simulink model "arm_stereo_ibvs_ekf_v1"  (R2025b)
settings: Solver=FixedStepDiscrete  StartTime=0  StopTime=inf  FixedStep=cfg.Ts  RelTol=1e-3
InitFcn:
  | init_arm_stereo_ibvs_ekf_v1
values from neighbouring files (symbols this model uses):
  cfg = cfgOverrideLocal    [init_arm_stereo_ibvs_ekf_v1.m]
  data = Stateflow.Data(chart)    [build_arm_stereo_ibvs_ekf_v1.m]
undefined symbols (not defined in the file or in its folder): cfg_armDepthRampTime, cfg_baseline, cfg_betaC, cfg_betaRho, cfg_cartesianLinearSpeedMax, cfg_cxL, cfg_cxR, cfg_cyL, cfg_cyR, cfg_disparityMin, cfg_disturbanceConfirmTime, cfg_ekfCovarianceJitter, cfg_ekfP0, cfg_ekfSConditionMin, cfg_ekfX0, cfg_epsilonC, cfg_epsilonRho, cfg_focalLength0Mm, cfg_focalLengthHardwareMaxMm, cfg_focalLengthHardwareMinMm, cfg_focalLengthWorkingMaxMm, cfg_focalLengthWorkingMinMm, cfg_focalRateAbsoluteMaxMmPerSec, cfg_focalRateGuaranteedMmPerSec, cfg_fr3Axis, cfg_fr3Joint8OriginRPY, cfg_fr3Joint8OriginXYZ, cfg_fr3OriginRPY, cfg_fr3OriginXYZ, cfg_imageWidth, cfg_Kc, cfg_kRho, cfg_lambdaC, cfg_lambdaRho, cfg_numericalEpsilon, cfg_outputPixelPitchXmm, cfg_outputPixelPitchYmm, cfg_p_CL_CR, cfg_pixelNoiseStd, cfg_q0, cfg_R_CL_CR, cfg_rhoMax, cfg_rhoMin, cfg_rightVisibilityHysteresisPx, cfg_rightVisibilityMarginPx, cfg_robustEnable, cfg_ros2InputTimeoutSec, cfg_scaleErrorEnterThreshold, cfg_scaleErrorExitThreshold, cfg_scaleSettledHoldTime, cfg_sigmaJerk, cfg_T_CL_CR, cfg_T_link8_CL, cfg_T_W_B, cfg_targetCharacteristicSize, cfg_Ts, cfg_visibilityEpsilon, cfg_visibilityZMin, cfg_zoomLimitMarginFraction, cfg_zoomOnlyMaxTime ... (+2)
libraries: ros2lib x7
(part 2 of 2)

== matlab function arm_stereo_ibvs_ekf_v1/Arm Priority Controller/MATLAB Function ==
  data: cameraVelocityCmd output; cLMeasured input; rhoHatL input; vHatLeft input; cLd input; rhoD input; validLeft input; ekfPredictionValid input; centerEnable input; depthEnable input; armEnable input; depthTaskWeight input; centerError output; depthError output; centerConditionMetric output; depthAuthority output; cameraVelocityCenter output; cameraVelocityDepthRaw output; cameraVelocityDepthWeighted output; cfg_numericalEpsilon parameter double size=[1 1]; cfg_robustEnable parameter double size=[1 1]; cfg_betaC parameter double size=[1 1]; cfg_epsilonC parameter double size=[1 1]; cfg_Kc parameter double size=[2 2]; cfg_lambdaC parameter double size=[1 1]; cfg_betaRho parameter double size=[1 1]; cfg_epsilonRho parameter double size=[1 1]; cfg_kRho parameter double size=[1 1]; cfg_lambdaRho parameter double size=[1 1]
function [cameraVelocityCmd, ...
          centerError, ...
          depthError, ...
          centerConditionMetric, ...
          depthAuthority, ...
          cameraVelocityCenter, ...
          cameraVelocityDepthRaw, ...
          cameraVelocityDepthWeighted] = fcn( ...
          cLMeasured, ...
          rhoHatL, ...
          vHatLeft, ...
          cLd, ...
          rhoD, ...
          validLeft, ...
          ekfPredictionValid, ...
          centerEnable, ...
          depthEnable, ...
          armEnable, ...
          depthTaskWeight, ...
          cfg_numericalEpsilon, ...
          cfg_robustEnable, ...
          cfg_betaC, ...
          cfg_epsilonC, ...
          cfg_Kc, ...
          cfg_lambdaC, ...
          cfg_betaRho, ...
          cfg_epsilonRho, ...
          cfg_kRho, ...
          cfg_lambdaRho)
%#codegen
% 输出均为左相机坐标系下的6维相机速度：
% [vx; vy; vz; wx; wy; wz]
%
% 中心任务为主任务，逆深度任务在中心任务零空间中执行。
% 关节速度映射、关节零空间和关节安全由外部ROS节点负责。

cameraVelocityCmd           = zeros(6,1);
centerError                 = zeros(2,1);
depthError                  = 0;
centerConditionMetric       = 0;
depthAuthority              = 0;
cameraVelocityCenter        = zeros(6,1);
cameraVelocityDepthRaw      = zeros(6,1);
cameraVelocityDepthWeighted = zeros(6,1);

%% 1. 基本安全门控
if armEnable <= 0.5 || validLeft <= 0.5
    return;
end

x = cLMeasured(1);
y = cLMeasured(2);

if ~isfinite(x) || ~isfinite(y)
    return;
end

%% 2. 选择逆深度和目标速度前馈
rho = max(rhoD, cfg_numericalEpsilon);
vFeed = zeros(3,1);

if ekfPredictionValid > 0.5 && ...
        isfinite(rhoHatL) && rhoHatL > cfg_numericalEpsilon && ...
        all(isfinite(vHatLeft))

    rho = max(rhoHatL, cfg_numericalEpsilon);
    vFeed = vHatLeft;
end

%% 3. 左相机中心任务
centerError = [x; y] - cLd;

Lc = [ ...
    -rho,  0,     x*rho, x*y,     -(1+x*x),  y;
     0,   -rho,   y*rho, 1+y*y,   -x*y,     -x];

Hc = rho * [ ...
    1, 0, -x;
    0, 1, -y];

bHatC = Hc * vFeed;

robustCenter = zeros(2,1);

if cfg_robustEnable > 0.5
    robustCenter = cfg_betaC * centerError / ...
        (sqrt(centerError' * centerError) + cfg_epsilonC);
end

nuCenter = -cfg_Kc * centerError ...
           -bHatC ...
           -robustCenter;

Gc = Lc * Lc' + cfg_lambdaC^2 * eye(2);
LcDampedInverse = Lc' / Gc;

cameraVelocityCenter = LcDampedInverse * nuCenter;

% 中心任务零空间
Ncenter = eye(6) - LcDampedInverse * Lc;

% 仅作为诊断值，越接近0说明中心任务数值条件越差
centerConditionMetric = det(Gc) / ...
    (trace(Gc)^2 + cfg_numericalEpsilon);

%% 4. 逆深度任务
depthError = rho - rhoD;

Lrho = [0, 0, rho*rho, rho*y, -rho*x, 0];
Hrho = [0, 0, -rho*rho];

bHatRho = Hrho * vFeed;

robustDepth = 0;

if cfg_robustEnable > 0.5
    robustDepth = cfg_betaRho * depthError / ...
        (abs(depthError) + cfg_epsilonRho);
end

nuDepth = -cfg_kRho * depthError ...
          -bHatRho ...
          -robustDepth;

% 深度任务在中心任务零空间中的有效方向
Adepth = Lrho * Ncenter;

depthAuthority = Adepth * Adepth';
depthDenominator = depthAuthority + cfg_lambdaRho^2;

depthWeight = min(max(depthTaskWeight, 0), 1);

if ekfPredictionValid <= 0.5
    depthWeight = 0;
end

cameraVelocityDepthRaw = ...
    Ncenter * Adepth' * ...
    ((nuDepth - Lrho * cameraVelocityCenter) / depthDenominator);

cameraVelocityDepthWeighted = ...
    depthWeight * cameraVelocityDepthRaw;

%% 5. 组合控制命令
if centerEnable > 0.5
    cameraVelocityCmd = cameraVelocityCenter;
end

if depthEnable > 0.5 && ekfPredictionValid > 0.5

    if centerEnable > 0.5
        % 中心主任务 + 深度零空间次任务
        cameraVelocityCmd = ...
            cameraVelocityCenter + cameraVelocityDepthWeighted;
    else
        % 仅执行深度任务
        standaloneDenominator = ...
            Lrho * Lrho' + cfg_lambdaRho^2;

        cameraVelocityDepthRaw = ...
            Lrho' * (nuDepth / standaloneDenominator);

        cameraVelocityDepthWeighted = ...
            depthWeight * cameraVelocityDepthRaw;

        cameraVelocityCenter = zeros(6,1);
        cameraVelocityCmd = cameraVelocityDepthWeighted;
    end
end

%% 6. 数值安全
if any(~isfinite(cameraVelocityCmd))
    cameraVelocityCmd = zeros(6,1);
end

if any(~isfinite(cameraVelocityCenter))
    cameraVelocityCenter = zeros(6,1);
end

if any(~isfinite(cameraVelocityDepthRaw))
    cameraVelocityDepthRaw = zeros(6,1);
end

if any(~isfinite(cameraVelocityDepthWeighted))
    cameraVelocityDepthWeighted = zeros(6,1);
end
end

== matlab function arm_stereo_ibvs_ekf_v1/Estimated Rho Dynamics/MATLAB Function ==
  data: normalizedFeatureMeasured input; rhoDotHat output; rhoHat input; vHatCL input; vHatCR input; JL input; JR input; qDotApplied input; cfg_R_CL_CR parameter double size=[3 3]; cfg_p_CL_CR parameter double size=[3 1]; cfg_numericalEpsilon parameter double size=[1 1]
function rhoDotHat = fcn(normalizedFeatureMeasured,rhoHat,vHatCL,vHatCR,JL,JR,qDotApplied, cfg_R_CL_CR, cfg_p_CL_CR, cfg_numericalEpsilon)
%#codegen
% Predicted inverse-depth rate from the applied left-camera twist.
rhoDotHat=zeros(2,1);
VCL=reshape(qDotApplied,6,1); R=cfg_R_CL_CR; p=cfg_p_CL_CR; S=[0 -p(3) p(2);p(3) 0 -p(1);-p(2) p(1) 0]; VCR=[R' -R'*S;zeros(3,3) R']*VCL;
for i=1:2
    if i==1, x=normalizedFeatureMeasured(1); y=normalizedFeatureMeasured(2); rho=max(rhoHat,cfg_numericalEpsilon); Vcam=VCL; vt=vHatCL;
    else, x=normalizedFeatureMeasured(3); y=normalizedFeatureMeasured(4); rho=max(rhoHat,cfg_numericalEpsilon); Vcam=VCR; vt=vHatCR; end
    Lrho=[0 0 rho*rho rho*y -rho*x 0]; Hrho=[0 0 -rho*rho];
    rhoDotHat(i)=Lrho*Vcam+Hrho*vt;
end
rhoDotHat=rhoDotHat+0*sum(JL(:))+0*sum(JR(:));
if any(~isfinite(rhoDotHat)), rhoDotHat=zeros(2,1); end
end

== matlab function arm_stereo_ibvs_ekf_v1/Right Visibility Guard/MATLAB Function ==
  data: xLeftMeasured input; uRightPredicted output; rhoHatSafe input; focalLengthMeasuredMm input; validLeft input; validRight input; ekfPredictionValid input; rightReacquireActive input; scaleDesiredNominal input; reset input; rightVisibilityMarginActualPx output; fRightMaxVisibleMm output; fRightMaxEffectiveMm output; rightScaleDesiredEffective output; rightVisibilityActive output; rightVisibilityInfeasible output; scaleDesiredEffective output; rightScaleDesiredNominal output; fRightMeasuredMm output; cfg_numericalEpsilon parameter double size=[1 1]; cfg_baseline parameter double size=[1 1]; cfg_outputPixelPitchXmm parameter double size=[1 1]; cfg_cxR parameter double size=[1 1]; cfg_imageWidth parameter double size=[1 1]; cfg_focalLengthHardwareMaxMm parameter double size=[2 1]; cfg_visibilityEpsilon parameter double size=[1 1]; cfg_rightVisibilityMarginPx parameter double size=[1 1]; cfg_focalLengthWorkingMaxMm parameter double size=[2 1]; cfg_focalLengthWorkingMinMm parameter double size=[2 1]; cfg_targetCharacteristicSize parameter double size=[1 1]; cfg_rightVisibilityHysteresisPx parameter double size=[1 1]
function [uRightPredicted,rightVisibilityMarginActualPx,fRightMaxVisibleMm,fRightMaxEffectiveMm,rightScaleDesiredEffective,rightVisibilityActive,rightVisibilityInfeasible,scaleDesiredEffective,rightScaleDesiredNominal,fRightMeasuredMm] = fcn(xLeftMeasured,rhoHatSafe,focalLengthMeasuredMm,validLeft,validRight,ekfPredictionValid,rightReacquireActive,scaleDesiredNominal,reset, cfg_numericalEpsilon, cfg_baseline, cfg_outputPixelPitchXmm, cfg_cxR, cfg_imageWidth, cfg_focalLengthHardwareMaxMm, cfg_visibilityEpsilon, cfg_rightVisibilityMarginPx, cfg_focalLengthWorkingMaxMm, cfg_focalLengthWorkingMinMm, cfg_targetCharacteristicSize, cfg_rightVisibilityHysteresisPx)
%#codegen
% CURRENT_STATE_VISIBILITY_GUARD; interface retained for future one-step prediction.
persistent active
if isempty(active), active=1; end
if reset>0.5, active=1; end
rightScaleDesiredNominal=scaleDesiredNominal(2); fRightMeasuredMm=focalLengthMeasuredMm(2); rho=max(rhoHatSafe,cfg_numericalEpsilon); xR=xLeftMeasured-cfg_baseline*rho; fRightPx=focalLengthMeasuredMm(2)/cfg_outputPixelPitchXmm;
uRightPredicted=cfg_cxR+fRightPx*xR; rightVisibilityMarginActualPx=min(uRightPredicted,cfg_imageWidth-uRightPredicted);
hardwareMaxPx=cfg_focalLengthHardwareMaxMm(2)/cfg_outputPixelPitchXmm;
if xR < -cfg_visibilityEpsilon, fMaxPx=(cfg_cxR-cfg_rightVisibilityMarginPx)/(-xR); elseif xR > cfg_visibilityEpsilon, fMaxPx=(cfg_imageWidth-cfg_rightVisibilityMarginPx-cfg_cxR)/xR; else, fMaxPx=hardwareMaxPx; end
fMaxPx=max(fMaxPx,0); fRightMaxVisibleMm=fMaxPx*cfg_outputPixelPitchXmm; rawEffective=min([cfg_focalLengthWorkingMaxMm(2);cfg_focalLengthHardwareMaxMm(2);fRightMaxVisibleMm]);
rightVisibilityInfeasible=double(rawEffective<cfg_focalLengthWorkingMinMm(2)); fRightMaxEffectiveMm=max(cfg_focalLengthWorkingMinMm(2),rawEffective);
scaleRightMaxVisible=cfg_targetCharacteristicSize*fMaxPx*rho; rightScaleDesiredEffective=min(scaleDesiredNominal(2),max(scaleRightMaxVisible,cfg_numericalEpsilon)); scaleDesiredEffective=[scaleDesiredNominal(1);rightScaleDesiredEffective];
enter=(validLeft<=0.5)||(ekfPredictionValid<=0.5)||(validRight<=0.5)||(rightReacquireActive>0.5)||(rightVisibilityInfeasible>0.5)||(uRightPredicted<cfg_rightVisibilityMarginPx)||(uRightPredicted>cfg_imageWidth-cfg_rightVisibilityMarginPx)||(focalLengthMeasuredMm(2)>fRightMaxEffectiveMm+cfg_numericalEpsilon);
exitOK=validLeft>0.5&&validRight>0.5&&ekfPredictionValid>0.5&&rightReacquireActive<=0.5&&rightVisibilityInfeasible<=0.5&&uRightPredicted>=cfg_rightVisibilityMarginPx+cfg_rightVisibilityHysteresisPx&&uRightPredicted<=cfg_imageWidth-cfg_rightVisibilityMarginPx-cfg_rightVisibilityHysteresisPx&&focalLengthMeasuredMm(2)<=fRightMaxEffectiveMm;
if enter, active=1; elseif exitOK, active=0; end; rightVisibilityActive=double(active>0.5);
if any(~isfinite([uRightPredicted;rightVisibilityMarginActualPx;fRightMaxVisibleMm;fRightMaxEffectiveMm;rightScaleDesiredEffective])), uRightPredicted=cfg_cxR; rightVisibilityMarginActualPx=0; fRightMaxVisibleMm=0; fRightMaxEffectiveMm=cfg_focalLengthWorkingMinMm(2); rightScaleDesiredEffective=cfg_numericalEpsilon; scaleDesiredEffective=[scaleDesiredNominal(1);rightScaleDesiredEffective]; rightVisibilityActive=1; rightVisibilityInfeasible=1; end
end

== matlab function arm_stereo_ibvs_ekf_v1/Zoom Controller/MATLAB Function ==
  data: fMeasuredMm input; fDotMmCmd output; scaleMeasured input; rhoHat input; rhoDotHat input; scaleDesiredEffective input; validLeft input; ekfPredictionValid input; focalAtWorkingLowerLimit input; focalAtWorkingUpperLimit input; fRightMaxEffectiveMm input; rightVisibilityActive input; rightReacquireActive input; fDotMmLimited output; scaleError output; gDotCmd output; focalCommandOutwardAtWorkingLimit output; focalFeasible output; focalRateUsageGuaranteedCmd output; focalRateUsageHardCmd output; cfg_focalLengthWorkingMaxMm parameter double size=[2 1]; cfg_numericalEpsilon parameter double size=[1 1]; cfg_robustEnable parameter double size=[1 1]; cfg_betaF parameter double size=[2 1]; cfg_epsilonF parameter double size=[2 1]; cfg_Kf parameter double size=[2 2]; cfg_targetCharacteristicSize parameter double size=[1 1]; cfg_outputPixelPitchXmm parameter double size=[1 1]; cfg_focalLengthWorkingMinMm parameter double size=[2 1]; cfg_rightReacquireZoomRateMmPerSec parameter double size=[1 1]; cfg_focalRateDesignMmPerSec parameter double size=[1 1]; cfg_Ts parameter double size=[1 1]; cfg_focalRateGuaranteedMmPerSec parameter double size=[1 1]; cfg_focalRateAbsoluteMaxMmPerSec parameter double size=[1 1]; cfg_zoomControlEnable parameter double size=[1 1]
function [fDotMmCmd,fDotMmLimited,scaleError,gDotCmd,focalCommandOutwardAtWorkingLimit,focalFeasible,focalRateUsageGuaranteedCmd,focalRateUsageHardCmd] = fcn(fMeasuredMm,scaleMeasured,rhoHat,rhoDotHat,scaleDesiredEffective,validLeft,ekfPredictionValid,focalAtWorkingLowerLimit,focalAtWorkingUpperLimit,fRightMaxEffectiveMm,rightVisibilityActive,rightReacquireActive, cfg_focalLengthWorkingMaxMm, cfg_numericalEpsilon, cfg_robustEnable, cfg_betaF, cfg_epsilonF, cfg_Kf, cfg_targetCharacteristicSize, cfg_outputPixelPitchXmm, cfg_focalLengthWorkingMinMm, cfg_rightReacquireZoomRateMmPerSec, cfg_focalRateDesignMmPerSec, cfg_Ts, cfg_focalRateGuaranteedMmPerSec, cfg_focalRateAbsoluteMaxMmPerSec, cfg_zoomControlEnable)
%#codegen
% Independent log-focal-length control; focal length is measured, not estimated.
fDotMmCmd=zeros(2,1); fDotMmLimited=zeros(2,1); scaleError=zeros(2,1); gDotCmd=zeros(2,1); focalCommandOutwardAtWorkingLimit=zeros(2,1); focalFeasible=ones(2,1); focalRateUsageGuaranteedCmd=zeros(2,1); focalRateUsageHardCmd=zeros(2,1);
upperEffective=[cfg_focalLengthWorkingMaxMm(1);fRightMaxEffectiveMm]; rho=max(rhoHat,cfg_numericalEpsilon);
for i=1:2
    r=max(scaleMeasured(i),cfg_numericalEpsilon); rd=max(scaleDesiredEffective(i),cfg_numericalEpsilon);
    scaleError(i)=log(r/rd); dHat=rhoDotHat(i)/rho; rf=0;
    if cfg_robustEnable>0.5, rf=cfg_betaF(i)*scaleError(i)/(abs(scaleError(i))+cfg_epsilonF(i)); end
    gDotCmd(i)=-cfg_Kf(i,i)*scaleError(i)-dHat-rf; fDotMmCmd(i)=fMeasuredMm(i)*gDotCmd(i);
    fRequiredMm=scaleDesiredEffective(i)/(cfg_targetCharacteristicSize*rho)*cfg_outputPixelPitchXmm; if fRequiredMm<cfg_focalLengthWorkingMinMm(i)||fRequiredMm>upperEffective(i), focalFeasible(i)=0; end
    focalCommandOutwardAtWorkingLimit(i)=double((focalAtWorkingLowerLimit(i)>0.5&&fDotMmCmd(i)<0)||(focalAtWorkingUpperLimit(i)>0.5&&fDotMmCmd(i)>0)||(fMeasuredMm(i)>=upperEffective(i)&&fDotMmCmd(i)>0));
end
if rightVisibilityActive>0.5||rightReacquireActive>0.5, if fMeasuredMm(2)>fRightMaxEffectiveMm+cfg_numericalEpsilon, fDotMmCmd(2)=-cfg_rightReacquireZoomRateMmPerSec; else, fDotMmCmd(2)=min(fDotMmCmd(2),0); end; end
if validLeft<=0.5||ekfPredictionValid<=0.5, fDotMmCmd(1)=0; if fMeasuredMm(1)>cfg_focalLengthWorkingMinMm(1), fDotMmCmd(1)=-cfg_rightReacquireZoomRateMmPerSec; end; fDotMmCmd(2)=0; if fMeasuredMm(2)>cfg_focalLengthWorkingMinMm(2), fDotMmCmd(2)=-cfg_rightReacquireZoomRateMmPerSec; end; end
fDotMmLimited=min(max(fDotMmCmd,-cfg_focalRateDesignMmPerSec),cfg_focalRateDesignMmPerSec); nextRight=fMeasuredMm(2)+cfg_Ts*fDotMmLimited(2); if fMeasuredMm(2)<=fRightMaxEffectiveMm&&nextRight>fRightMaxEffectiveMm, fDotMmLimited(2)=min(fDotMmLimited(2),(fRightMaxEffectiveMm-fMeasuredMm(2))/cfg_Ts); end
focalRateUsageGuaranteedCmd=abs(fDotMmLimited)/cfg_focalRateGuaranteedMmPerSec; focalRateUsageHardCmd=abs(fDotMmLimited)/cfg_focalRateAbsoluteMaxMmPerSec;
if cfg_zoomControlEnable<=0.5 || any(~isfinite(fDotMmCmd))||any(~isfinite(fDotMmLimited)), fDotMmCmd=zeros(2,1); fDotMmLimited=zeros(2,1); gDotCmd=zeros(2,1); focalRateUsageGuaranteedCmd=zeros(2,1); focalRateUsageHardCmd=zeros(2,1); end
end

== matlab function arm_stereo_ibvs_ekf_v1/Zoom Priority Supervisor/MATLAB Function ==
  data: scaleError input; depthTaskWeight output; depthError input; focalLengthMeasuredMm input; focalAtWorkingLowerLimit input; focalAtWorkingUpperLimit input; focalHeadroomMm input; focalFeasible input; validLeft input; validStereoQualified input; ekfPredictionValid input; reset input; focalCommandOutwardAtWorkingLimit input; focalRateUsageGuaranteed input; focalRateUsageHard input; rightReacquireActive input; schedulerMode output; zoomPriorityActive output; zoomPriorityTimer output; scaleSettledTimer output; armRecoveryReason output; newDisturbanceDetected output; cfg_zoomPriorityEnable parameter double size=[1 1]; cfg_armDepthRampTime parameter double size=[1 1]; cfg_scaleErrorEnterThreshold parameter double size=[1 1]; cfg_Ts parameter double size=[1 1]; cfg_scaleErrorExitThreshold parameter double size=[1 1]; cfg_disturbanceConfirmTime parameter double size=[1 1]; cfg_scaleSettledHoldTime parameter double size=[1 1]; cfg_zoomOnlyMaxTime parameter double size=[1 1]
function [depthTaskWeight,schedulerMode,zoomPriorityActive,zoomPriorityTimer,scaleSettledTimer,armRecoveryReason,newDisturbanceDetected]=fcn(scaleError,depthError,focalLengthMeasuredMm,focalAtWorkingLowerLimit,focalAtWorkingUpperLimit,focalHeadroomMm,focalFeasible,validLeft,validStereoQualified,ekfPredictionValid,reset,focalCommandOutwardAtWorkingLimit,focalRateUsageGuaranteed,focalRateUsageHard,rightReacquireActive, cfg_zoomPriorityEnable, cfg_armDepthRampTime, cfg_scaleErrorEnterThreshold, cfg_Ts, cfg_scaleErrorExitThreshold, cfg_disturbanceConfirmTime, cfg_scaleSettledHoldTime, cfg_zoomOnlyMaxTime)
%#codegen
% Modes: 0 INITIALIZE, 1 ZOOM_FIRST, 2 ARM_RECOVERY, 3 FULL_TRACK, 4 SAFE_HOLD, 5 RIGHT_REACQUIRE.
persistent mode zoomTimer settledTimer rampTimer reason disturbanceTimer validLast rateTimer
if isempty(mode), mode=0; zoomTimer=0; settledTimer=0; rampTimer=0; reason=0; disturbanceTimer=0; validLast=0; rateTimer=0; end
if reset>0.5, mode=0; zoomTimer=0; settledTimer=0; rampTimer=0; reason=0; disturbanceTimer=0; validLast=0; rateTimer=0; end
depthTaskWeight=0; newDisturbanceDetected=0; centerValid=validLeft>0.5; depthReady=validStereoQualified>0.5&&ekfPredictionValid>0.5&&rightReacquireActive<=0.5; e=max(abs(scaleError));
if ~centerValid, mode=4; depthTaskWeight=0; validLast=0;
elseif ~depthReady, mode=5; depthTaskWeight=0; validLast=0; rampTimer=0;
elseif cfg_zoomPriorityEnable<=0.5, mode=3; depthTaskWeight=1; zoomTimer=0; settledTimer=0; rampTimer=cfg_armDepthRampTime; reason=0; disturbanceTimer=0; validLast=1;
else
    if validLast<0.5&&(mode==4||mode==5), mode=1; zoomTimer=0; settledTimer=0; rampTimer=0; reason=0; disturbanceTimer=0; end
    if mode==0, if e>cfg_scaleErrorEnterThreshold, mode=1; depthTaskWeight=0; else, mode=3; depthTaskWeight=1; end
    elseif mode==1
        depthTaskWeight=0; zoomTimer=zoomTimer+cfg_Ts; if e<=cfg_scaleErrorExitThreshold, settledTimer=settledTimer+cfg_Ts; else, settledTimer=0; end
        if any(focalRateUsageGuaranteed>=1), rateTimer=rateTimer+cfg_Ts; else, rateTimer=0; end
        if any(focalRateUsageHard>=1), mode=2; reason=6; rampTimer=0;
        elseif rateTimer>=cfg_disturbanceConfirmTime&&e>cfg_scaleErrorExitThreshold, mode=2; reason=5; rampTimer=0;
        elseif settledTimer>=cfg_scaleSettledHoldTime, mode=2; reason=1; rampTimer=0;
        elseif any(focalCommandOutwardAtWorkingLimit>0.5), mode=2; reason=7; rampTimer=0;
        elseif zoomTimer>=cfg_disturbanceConfirmTime&&any(focalFeasible<0.5), mode=2; reason=3; rampTimer=0;
        elseif zoomTimer>=cfg_zoomOnlyMaxTime, mode=2; reason=4; rampTimer=0; end
    elseif mode==2
        rampTimer=min(rampTimer+cfg_Ts,cfg_armDepthRampTime); s=min(max(rampTimer/max(cfg_armDepthRampTime,cfg_Ts),0),1); depthTaskWeight=s*s*(3-2*s); if depthTaskWeight>=1-1e-6, mode=3; depthTaskWeight=1; disturbanceTimer=0; end
    elseif mode==3
        depthTaskWeight=1; if e>=cfg_scaleErrorEnterThreshold, depthTaskWeight=0; disturbanceTimer=disturbanceTimer+cfg_Ts; else, disturbanceTimer=0; end
        if disturbanceTimer>=cfg_disturbanceConfirmTime, mode=1; depthTaskWeight=0; zoomTimer=0; settledTimer=0; rampTimer=0; reason=0; disturbanceTimer=0; newDisturbanceDetected=1; end
    else, mode=1; depthTaskWeight=0; zoomTimer=0; settledTimer=0; rampTimer=0; reason=0; end
    validLast=1;
end
schedulerMode=mode; zoomPriorityActive=double(mode==1); zoomPriorityTimer=zoomTimer; scaleSettledTimer=settledTimer; armRecoveryReason=reason;
if any(~isfinite([depthTaskWeight;schedulerMode;zoomPriorityTimer;scaleSettledTimer;depthError;focalLengthMeasuredMm;focalHeadroomMm;focalAtWorkingLowerLimit;focalAtWorkingUpperLimit])), depthTaskWeight=0; schedulerMode=4; zoomPriorityActive=0; newDisturbanceDetected=0; end
end

== matlab function arm_stereo_ibvs_ekf_v1/Zoom Safety and Saturation/MATLAB Function ==
  data: cameraVelocityCmd input; cameraVelocityApplied output; fDotMmLimited input; focalLengthMeasuredMm input; validLeft input; armEnable input; cfg_cartesianLinearSpeedMax parameter double size=[1 1]; cfg_cartesianAngularSpeedMax input; cfg_focalRateAbsoluteMaxMmPerSec parameter double size=[1 1]; cfg_focalLengthWorkingMinMm parameter double size=[2 1]; cfg_focalLengthWorkingMaxMm parameter double size=[2 1]; cfg_focalLengthHardwareMinMm parameter double size=[2 1]; cfg_focalLengthHardwareMaxMm parameter double size=[2 1]; cfg_Ts parameter double size=[1 1]; cfg_focalRateGuaranteedMmPerSec parameter double size=[1 1]; fDotMmApplied output; cameraVelocitySaturationFlag output; focalRateSaturationFlag output; linearSpeed output; angularSpeed output; linearSpeedScale output; angularSpeedScale output; linearSpeedSaturationFlag output; angularSpeedSaturationFlag output; focalBoundaryWarning output; focalLengthCommandMm output; focalRateUsageGuaranteed output; focalRateUsageHard output; focalRateHardViolation output; cfg_numericalEpsilon parameter double size=[7 1]
function [cameraVelocityApplied, ...
          fDotMmApplied, ...
          cameraVelocitySaturationFlag, ...
          focalRateSaturationFlag, ...
          linearSpeed, ...
          angularSpeed, ...
          linearSpeedScale, ...
          angularSpeedScale, ...
          linearSpeedSaturationFlag, ...
          angularSpeedSaturationFlag, ...
          focalBoundaryWarning, ...
          focalLengthCommandMm, ...
          focalRateUsageGuaranteed, ...
          focalRateUsageHard, ...
          focalRateHardViolation] = fcn( ...
          cameraVelocityCmd, ...
          fDotMmLimited, ...
          focalLengthMeasuredMm, ...
          validLeft, ...
          armEnable, ...
          cfg_cartesianLinearSpeedMax, ...
          cfg_cartesianAngularSpeedMax, ...
          cfg_focalRateAbsoluteMaxMmPerSec, ...
          cfg_focalLengthWorkingMinMm, ...
          cfg_focalLengthWorkingMaxMm, ...
          cfg_focalLengthHardwareMinMm, ...
          cfg_focalLengthHardwareMaxMm, ...
          cfg_Ts, ...
          cfg_focalRateGuaranteedMmPerSec, ...
          cfg_numericalEpsilon)
%#codegen
% ROS部署版安全模块。
%
% cameraVelocityCmd:
% 左相机坐标系中的6维速度
% [vx; vy; vz; wx; wy; wz]
%
% 本模块只处理：
% 1. 相机线速度限制
% 2. 相机角速度限制
% 3. 焦距速度限制
% 4. 焦距工作范围和硬件范围保护
%
% 关节速度、关节限位、关节加速度和奇异性保护
% 由外部Python/C++关节速度映射节点负责。

cameraVelocityApplied = zeros(6,1);
fDotMmApplied = zeros(2,1);

cameraVelocitySaturationFlag = 0;
focalRateSaturationFlag = 0;

linearSpeed = 0;
angularSpeed = 0;

linearSpeedScale = 1;
angularSpeedScale = 1;

linearSpeedSaturationFlag = 0;
angularSpeedSaturationFlag = 0;

focalBoundaryWarning = zeros(2,1);

focalLengthCommandMm = zeros(2,1);
focalRateUsageGuaranteed = zeros(2,1);
focalRateUsageHard = zeros(2,1);
focalRateHardViolation = zeros(2,1);

%% 1. 相机速度安全限制

cameraCommandFinite = all(isfinite(cameraVelocityCmd));

if validLeft > 0.5 && ...
        armEnable > 0.5 && ...
        cameraCommandFinite

    linearVelocity = cameraVelocityCmd(1:3);
    angularVelocity = cameraVelocityCmd(4:6);

    linearSpeedRaw = norm(linearVelocity);
    angularSpeedRaw = norm(angularVelocity);

    linearSpeed = linearSpeedRaw;
    angularSpeed = angularSpeedRaw;

    linearLimit = max( ...
        cfg_cartesianLinearSpeedMax, ...
        cfg_numericalEpsilon);

    angularLimit = max( ...
        cfg_cartesianAngularSpeedMax, ...
        cfg_numericalEpsilon);

    % 线速度整体等比例缩放
    if linearSpeedRaw > linearLimit
        linearSpeedScale = linearLimit / linearSpeedRaw;
        linearVelocity = linearSpeedScale * linearVelocity;

        linearSpeed = linearLimit;
        linearSpeedSaturationFlag = 1;
    end

    % 角速度整体等比例缩放
    if angularSpeedRaw > angularLimit
        angularSpeedScale = angularLimit / angularSpeedRaw;
        angularVelocity = angularSpeedScale * angularVelocity;

        angularSpeed = angularLimit;
        angularSpeedSaturationFlag = 1;
    end

    cameraVelocityApplied = [ ...
        linearVelocity;
        angularVelocity];
end

if ~cameraCommandFinite
    cameraVelocityApplied = zeros(6,1);
    cameraVelocitySaturationFlag = 1;

elseif any(abs(cameraVelocityApplied-cameraVelocityCmd) > 1e-12)
    cameraVelocitySaturationFlag = 1;
end

if any(~isfinite(cameraVelocityApplied))
    cameraVelocityApplied = zeros(6,1);

    cameraVelocitySaturationFlag = 1;
    linearSpeed = 0;
    angularSpeed = 0;
    linearSpeedScale = 0;
    angularSpeedScale = 0;
end

%% 2. 焦距状态初始化

focalStateFinite = all(isfinite(focalLengthMeasuredMm));

if focalStateFinite
    focalLengthCommandMm = min( ...
        max(focalLengthMeasuredMm, ...
            cfg_focalLengthHardwareMinMm), ...
        cfg_focalLengthHardwareMaxMm);
end

%% 3. 焦距速度硬件限幅

focalRateLimit = max( ...
    cfg_focalRateAbsoluteMaxMmPerSec, ...
    cfg_numericalEpsilon);

if all(isfinite(fDotMmLimited)) && focalStateFinite

    focalRateHardViolation = double( ...
        abs(fDotMmLimited) > ...
        cfg_focalRateAbsoluteMaxMmPerSec);

    fDotMmApplied = min( ...
        max(fDotMmLimited, ...
            -cfg_focalRateAbsoluteMaxMmPerSec), ...
        cfg_focalRateAbsoluteMaxMmPerSec);

    %% 4. 焦距边界保护

    for i = 1:2

        currentFocal = focalLengthMeasuredMm(i);

        belowWorking = ...
            currentFocal <= cfg_focalLengthWorkingMinMm(i);

        aboveWorking = ...
            currentFocal >= cfg_focalLengthWorkingMaxMm(i);

        belowHardware = ...
            currentFocal <= cfg_focalLengthHardwareMinMm(i);

        aboveHardware = ...
            currentFocal >= cfg_focalLengthHardwareMaxMm(i);

        focalBoundaryWarning(i) = double( ...
            belowWorking || ...
            aboveWorking || ...
            belowHardware || ...
            aboveHardware);

        % 已经位于下边界，不允许继续减小焦距
        if (belowWorking || belowHardware) && ...
                fDotMmApplied(i) < 0

            fDotMmApplied(i) = 0;
        end

        % 已经位于上边界，不允许继续增大焦距
        if (aboveWorking || aboveHardware) && ...
                fDotMmApplied(i) > 0

            fDotMmApplied(i) = 0;
        end

        %% 预测下一采样周期的焦距

        nextFocal = currentFocal + ...
            cfg_Ts * fDotMmApplied(i);

        % 防止跨越工作下限
        if currentFocal >= ...
                cfg_focalLengthWorkingMinMm(i) && ...
                nextFocal < ...
                cfg_focalLengthWorkingMinMm(i)

            fDotMmApplied(i) = ...
                (cfg_focalLengthWorkingMinMm(i) ...
                -currentFocal) / cfg_Ts;
        end

        % 防止跨越工作上限
        if currentFocal <= ...
                cfg_focalLengthWorkingMaxMm(i) && ...
                nextFocal > ...
                cfg_focalLengthWorkingMaxMm(i)

            fDotMmApplied(i) = ...
                (cfg_focalLengthWorkingMaxMm(i) ...
                -currentFocal) / cfg_Ts;
        end

        % 再次预测
        nextFocal = currentFocal + ...
            cfg_Ts * fDotMmApplied(i);

        % 防止跨越硬件下限
        if currentFocal >= ...
                cfg_focalLengthHardwareMinMm(i) && ...
                nextFocal < ...
                cfg_focalLengthHardwareMinMm(i)

            fDotMmApplied(i) = ...
                (cfg_focalLengthHardwareMinMm(i) ...
                -currentFocal) / cfg_Ts;
        end

        % 防止跨越硬件上限
        if currentFocal <= ...
                cfg_focalLengthHardwareMaxMm(i) && ...
                nextFocal > ...
                cfg_focalLengthHardwareMaxMm(i)

            fDotMmApplied(i) = ...
                (cfg_focalLengthHardwareMaxMm(i) ...
                -currentFocal) / cfg_Ts;
        end
    end
else
    fDotMmApplied = zeros(2,1);
    focalRateSaturationFlag = 1;
end

%% 5. 焦距速度变化检查

if all(isfinite(fDotMmLimited))
    if any(abs(fDotMmApplied-fDotMmLimited) > 1e-12)
        focalRateSaturationFlag = 1;
    end
else
    focalRateSaturationFlag = 1;
end

if any(~isfinite(fDotMmApplied))
    fDotMmApplied = zeros(2,1);
    focalRateSaturationFlag = 1;
end

%% 6. 使用率与下一周期焦距

guaranteedRate = max( ...
    cfg_focalRateGuaranteedMmPerSec, ...
    cfg_numericalEpsilon);

focalRateUsageGuaranteed = ...
    abs(fDotMmApplied) / guaranteedRate;

focalRateUsageHard = ...
    abs(fDotMmApplied) / focalRateLimit;

if focalStateFinite
    focalLengthCommandMm = min( ...
        max( ...
            focalLengthMeasuredMm ...
            +cfg_Ts*fDotMmApplied, ...
            cfg_focalLengthHardwareMinMm), ...
        cfg_focalLengthHardwareMaxMm);
end
end

== matlab function arm_stereo_ibvs_ekf_v1/FR3 Camera Kinematics/MATLAB Function ==
  data: q input; pWCL output; RWCL output; pWCR output; RWCR output; JL output; JR output; rankJL output; rcondJL output; rotationOrthogonalityError output; baselineLength output; baselineError output; stereoRotationError output; pWLink8 output; RWLink8 output; cfg_T_W_B parameter double size=[4 4]; cfg_fr3OriginXYZ parameter double size=[3 7]; cfg_fr3OriginRPY parameter double size=[3 7]; cfg_fr3Axis parameter double size=[3 7]; cfg_fr3Joint8OriginXYZ parameter double size=[3 1]; cfg_fr3Joint8OriginRPY parameter double size=[3 1]; cfg_T_link8_CL parameter double size=[4 4]; cfg_T_CL_CR parameter double size=[4 4]; cfg_R_CL_CR parameter double size=[3 3]; cfg_p_CL_CR parameter double size=[3 1]
function [pWCL,RWCL,pWCR,RWCR,JL,JR,rankJL,rcondJL,rotationOrthogonalityError,baselineLength,baselineError,stereoRotationError,pWLink8,RWLink8] = fcn(q, cfg_T_W_B, cfg_fr3OriginXYZ, cfg_fr3OriginRPY, cfg_fr3Axis, cfg_fr3Joint8OriginXYZ, cfg_fr3Joint8OriginRPY, cfg_T_link8_CL, cfg_T_CL_CR, cfg_R_CL_CR, cfg_p_CL_CR)
%#codegen
% URDF-derived FK and optical-center Jacobians; no pose integration.
pWCL=zeros(3,1); RWCL=eye(3); pWCR=zeros(3,1); RWCR=eye(3); JL=zeros(6,7); JR=zeros(6,7); rankJL=0; rcondJL=0; rotationOrthogonalityError=0; baselineLength=0; baselineError=0; stereoRotationError=0; pWLink8=zeros(3,1); RWLink8=eye(3);
T=cfg_T_W_B; jointOrigins=zeros(3,7); jointAxes=zeros(3,7);
for i=1:7
    xyz=cfg_fr3OriginXYZ(:,i); rpy=cfg_fr3OriginRPY(:,i);
    cr=cos(rpy(1));sr=sin(rpy(1));cp=cos(rpy(2));sp=sin(rpy(2));cy=cos(rpy(3));sy=sin(rpy(3));
    Rx=[1 0 0;0 cr -sr;0 sr cr]; Ry=[cp 0 sp;0 1 0;-sp 0 cp]; Rz=[cy -sy 0;sy cy 0;0 0 1]; To=eye(4); To(1:3,1:3)=Rz*Ry*Rx; To(1:3,4)=xyz; T=T*To;
    jointOrigins(:,i)=T(1:3,4); axis=cfg_fr3Axis(:,i); jointAxes(:,i)=T(1:3,1:3)*axis;
    u=axis/max(norm(axis),eps); K=[0 -u(3) u(2);u(3) 0 -u(1);-u(2) u(1) 0]; Tr=eye(4); Tr(1:3,1:3)=eye(3)+sin(q(i))*K+(1-cos(q(i)))*(K*K); T=T*Tr;
end
xyz=cfg_fr3Joint8OriginXYZ; rpy=cfg_fr3Joint8OriginRPY; cr=cos(rpy(1));sr=sin(rpy(1));cp=cos(rpy(2));sp=sin(rpy(2));cy=cos(rpy(3));sy=sin(rpy(3)); Rx=[1 0 0;0 cr -sr;0 sr cr]; Ry=[cp 0 sp;0 1 0;-sp 0 cp]; Rz=[cy -sy 0;sy cy 0;0 0 1]; To=eye(4); To(1:3,1:3)=Rz*Ry*Rx; To(1:3,4)=xyz; T=T*To;
pWLink8=T(1:3,4); RWLink8=T(1:3,1:3); TCL=T*cfg_T_link8_CL; pWCL=TCL(1:3,4); RWCL=TCL(1:3,1:3); TCR=TCL*cfg_T_CL_CR; pWCR=TCR(1:3,4); RWCR=TCR(1:3,1:3);
JW=zeros(6,7); for i=1:7, JW(1:3,i)=cross(jointAxes(:,i),pWCL-jointOrigins(:,i)); JW(4:6,i)=jointAxes(:,i); end
RCLW=RWCL'; JL=[RCLW zeros(3,3);zeros(3,3) RCLW]*JW; R=cfg_R_CL_CR; p=cfg_p_CL_CR; S=[0 -p(3) p(2);p(3) 0 -p(1);-p(2) p(1) 0]; JR=[R' -R'*S;zeros(3,3) R']*JL;
rankJL=rank(JL); rcondJL=rcond(JL*JL'); rotationOrthogonalityError=norm(RWCL'*RWCL-eye(3),'fro'); baselineLength=norm(pWCR-pWCL); baselineError=abs(baselineLength-norm(cfg_p_CL_CR)); stereoRotationError=norm(RWCR-RWCL*cfg_R_CL_CR,'fro');
end

== matlab function arm_stereo_ibvs_ekf_v1/Focal State Calibration/MATLAB Function ==
  data: fMm input; focalLengthMeasuredMm output; fxMeasuredPx output; fyMeasuredPx output; focalAtWorkingLowerLimit output; focalAtWorkingUpperLimit output; focalAtHardwareLowerLimit output; focalAtHardwareUpperLimit output; focalOutsideWorkingRange output; focalHardwareLimitViolation output; focalRangeUsage output; focalHeadroomMm output; focalLengthWorkingMinMm output; focalLengthWorkingMaxMm output; focalLengthHardwareMinMm output; focalLengthHardwareMaxMm output; cfg_focalLengthHardwareMinMm parameter double size=[2 1]; cfg_focalLengthHardwareMaxMm parameter double size=[2 1]; cfg_outputPixelPitchXmm parameter double size=[1 1]; cfg_outputPixelPitchYmm parameter double size=[1 1]; cfg_focalLengthWorkingMaxMm parameter double size=[2 1]; cfg_focalLengthWorkingMinMm parameter double size=[2 1]; cfg_zoomLimitMarginFraction parameter double size=[1 1]; cfg_numericalEpsilon parameter double size=[1 1]
function [focalLengthMeasuredMm,fxMeasuredPx,fyMeasuredPx,focalAtWorkingLowerLimit,focalAtWorkingUpperLimit,focalAtHardwareLowerLimit,focalAtHardwareUpperLimit,focalOutsideWorkingRange,focalHardwareLimitViolation,focalRangeUsage,focalHeadroomMm,focalLengthWorkingMinMm,focalLengthWorkingMaxMm,focalLengthHardwareMinMm,focalLengthHardwareMaxMm]=fcn(fMm, cfg_focalLengthHardwareMinMm, cfg_focalLengthHardwareMaxMm, cfg_outputPixelPitchXmm, cfg_outputPixelPitchYmm, cfg_focalLengthWorkingMaxMm, cfg_focalLengthWorkingMinMm, cfg_zoomLimitMarginFraction, cfg_numericalEpsilon)
%#codegen
focalLengthMeasuredMm=min(max(fMm,cfg_focalLengthHardwareMinMm),cfg_focalLengthHardwareMaxMm);
fxMeasuredPx=focalLengthMeasuredMm/cfg_outputPixelPitchXmm; fyMeasuredPx=focalLengthMeasuredMm/cfg_outputPixelPitchYmm;
wspan=cfg_focalLengthWorkingMaxMm-cfg_focalLengthWorkingMinMm; hspan=cfg_focalLengthHardwareMaxMm-cfg_focalLengthHardwareMinMm; margin=cfg_zoomLimitMarginFraction*wspan;
focalAtWorkingLowerLimit=double(focalLengthMeasuredMm<=cfg_focalLengthWorkingMinMm+margin); focalAtWorkingUpperLimit=double(focalLengthMeasuredMm>=cfg_focalLengthWorkingMaxMm-margin);
focalAtHardwareLowerLimit=double(focalLengthMeasuredMm<=cfg_focalLengthHardwareMinMm+cfg_numericalEpsilon); focalAtHardwareUpperLimit=double(focalLengthMeasuredMm>=cfg_focalLengthHardwareMaxMm-cfg_numericalEpsilon);
focalOutsideWorkingRange=double(focalLengthMeasuredMm<cfg_focalLengthWorkingMinMm|focalLengthMeasuredMm>cfg_focalLengthWorkingMaxMm); focalHardwareLimitViolation=double(focalLengthMeasuredMm<cfg_focalLengthHardwareMinMm|focalLengthMeasuredMm>cfg_focalLengthHardwareMaxMm);
focalRangeUsage=(focalLengthMeasuredMm-cfg_focalLengthWorkingMinMm)./max(wspan,cfg_numericalEpsilon*ones(2,1)); focalHeadroomMm=min(focalLengthMeasuredMm-cfg_focalLengthWorkingMinMm,cfg_focalLengthWorkingMaxMm-focalLengthMeasuredMm);
focalLengthWorkingMinMm=cfg_focalLengthWorkingMinMm; focalLengthWorkingMaxMm=cfg_focalLengthWorkingMaxMm; focalLengthHardwareMinMm=cfg_focalLengthHardwareMinMm; focalLengthHardwareMaxMm=cfg_focalLengthHardwareMaxMm;
end

== matlab function arm_stereo_ibvs_ekf_v1/Camera Velocity Output/MATLAB Function ==
  data: cameraVelocityCmd input; cameraVelocity output; validLeft input; cfg_cartesianLinearSpeedMax parameter double size=[1 1]
function cameraVelocity=fcn(cameraVelocityCmd,validLeft, cfg_cartesianLinearSpeedMax)
%#codegen
cameraVelocity=zeros(6,1);
if validLeft>0.5 && all(isfinite(cameraVelocityCmd)), cameraVelocity=reshape(cameraVelocityCmd,6,1); end
linearSpeed=norm(cameraVelocity(1:3)); if linearSpeed>cfg_cartesianLinearSpeedMax, cameraVelocity=cameraVelocity*(cfg_cartesianLinearSpeedMax/linearSpeed); end
if any(~isfinite(cameraVelocity)), cameraVelocity=zeros(6,1); end
end

== matlab function arm_stereo_ibvs_ekf_v1/ROS Vision Decoder/MATLAB Function ==
  data: features input; pixelMeasurement output; isNew input; scaleMeasured output; validLeft output; validRight output; visionFresh output; cfg_Ts parameter double size=[1 1]; cfg_ros2InputTimeoutSec parameter double size=[1 1]
function [pixelMeasurement,scaleMeasured,validLeft,validRight,visionFresh]=fcn(features,isNew, cfg_Ts, cfg_ros2InputTimeoutSec)
%#codegen
persistent age last
if isempty(age), age=inf; last=zeros(8,1); end
if isNew, last=reshape(features,8,1); age=0; else, age=age+cfg_Ts; end
visionFresh=double(age<=cfg_ros2InputTimeoutSec);
validLeft=double(visionFresh>0.5 && last(1)>0.5); validRight=double(visionFresh>0.5 && last(2)>0.5);
pixelMeasurement=[last(3);last(4);last(5);last(6)]; scaleMeasured=[last(7);last(8)];
if any(~isfinite([pixelMeasurement;scaleMeasured])), pixelMeasurement=zeros(4,1); scaleMeasured=zeros(2,1); validLeft=0; validRight=0; end
end

== matlab function arm_stereo_ibvs_ekf_v1/ROS Joint Decoder/MATLAB Function ==
  data: position input; q output; isNew input; jointFresh output; cfg_q0 parameter double size=[7 1]; cfg_Ts parameter double size=[1 1]; cfg_ros2InputTimeoutSec parameter double size=[1 1]
function [q,jointFresh]=fcn(position,isNew, cfg_q0, cfg_Ts, cfg_ros2InputTimeoutSec)
%#codegen
persistent age last
if isempty(age), age=inf; last=cfg_q0; end
if isNew, candidate=reshape(position,7,1); if all(isfinite(candidate)), last=candidate; age=0; end, else, age=age+cfg_Ts; end
q=last; jointFresh=double(age<=cfg_ros2InputTimeoutSec);
end

== matlab function arm_stereo_ibvs_ekf_v1/ROS Focal Decoder/MATLAB Function ==
  data: focalMm input; focalLengthMeasuredMm output; isNew input; focalFresh output; cfg_focalLength0Mm parameter double size=[2 1]; cfg_Ts parameter double size=[1 1]; cfg_ros2InputTimeoutSec parameter double size=[1 1]
function [focalLengthMeasuredMm,focalFresh]=fcn(focalMm,isNew, cfg_focalLength0Mm, cfg_Ts, cfg_ros2InputTimeoutSec)
%#codegen
persistent age last
if isempty(age), age=inf; last=cfg_focalLength0Mm; end
if isNew, candidate=reshape(focalMm,2,1); if all(isfinite(candidate)) && all(candidate>0), last=candidate; age=0; end, else, age=age+cfg_Ts; end
focalLengthMeasuredMm=last; focalFresh=double(age<=cfg_ros2InputTimeoutSec);
end
